simulink model "gamma_hat"  (R2015b)
settings: Solver=VariableStepAuto  StartTime=0.0  StopTime=10.0  RelTol=1e-3
settings Model: Creator=yuji  LastModifiedBy=yuji

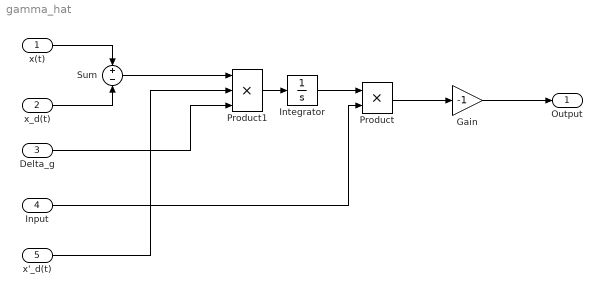
== system gamma_hat ==
  x(t) : Inport
  x_d(t) : Inport  Port=2
  Delta_g : Inport  Port=3
  Input : Inport  Port=4
  x'_d(t) : Inport  Port=5
  Gain : Gain  Gain=-1
  Integrator : Integrator
  Product : Product
  Product1 : Product  Inputs=3
  Sum : Sum  Inputs=+|-
  Output : Outport
  wires:
  x(t)/1 -> Sum/1
  x_d(t)/1 -> Sum/2
  Integrator/1 -> Product/1
  Input/1 -> Product/2
  Product1/1 -> Integrator/1
  Sum/1 -> Product1/1
  Delta_g/1 -> Product1/3
  Product/1 -> Gain/1
  Gain/1 -> Output/1
  x'_d(t)/1 -> Product1/2
